simulink model "PMSM_PI_decomposition2018b"  (R2020a)
settings: Solver=ode23tb  StartTime=0.0  StopTime=1  FixedStep=Ts  RelTol=1e-4  EnableMultiTasking=on
InitFcn:
  | Ts = 10e-6;
  | 
  | R = 0.958;
  | Ld = 5.25e-3;
  | Lq = 12e-3;
  | Pn = 4;
  | flux = 0.1827;
undefined symbols (not defined in the file or in its folder): DiscIntNeverNeededParam
libraries: powerlib x4, simulink x1
settings Model: Creator=SUN  LastModifiedBy=Lenovo
settings SolverCC: ZeroCrossControl=DisableAll
settings DataIOCC: LimitDataPoints=on  SaveFormat=Array  SignalLoggingSaveFormat=ModelDataLogs  ReturnWorkspaceOutputs=off
settings OptimizationCC: ExpressionDepthLimit=2147483647  InitFltsAndDblsToZero=on  LifeSpan=inf
settings DebuggingCC: UnderspecifiedInitializationDetection=Classic  MergeDetectMultiDrivingBlocksExec=none  SolverPrmCheckMsg=warning  FcnCallInpInsideContextMsg=warning  StateNameClashWarn=warning  SFUnexpectedBacktrackingDiag=warning  SFNoUnconditionalDefaultTransitionDiag=warning  SFExecutionAtInitializationDiag=none  ArithmeticOperatorsInVariantConditions=warning
settings HardwareCC: ProdBitPerPointer=32  ProdBitPerSizeT=32  ProdBitPerPtrDiffT=32  ProdLargestAtomicFloat=None  ProdIntDivRoundTo=Undefined  ProdEndianess=Unspecified  ProdWordSize=32  ProdHWDeviceType=32-bit Generic
settings ModelReferenceCC: PropagateSignalLabelsOutOfModel=off
settings SFSimCC: SimUseLocalCustomCode=off  CustomCodeUndefinedFunction=UseInterfaceOnly
settings RTWCC: RTWUseLocalCustomCode=off
settings CodeAppCC: StateflowObjectComments=on
settings GRTTargetCC: TargetLangStandard=C89/C90 (ANSI)  CombineOutputUpdateFcns=off  GRTInterface=on
settings ConfigComp: CovMetricSettings=dw  CovHtmlReporting=on  CovSaveCumulativeToWorkspaceVar=on  CovSaveSingleToWorkspaceVar=on  CovExternalEMLEnable=off  CovSFcnEnable=off
settings SimscapeCC: SimscapeNormalizeSystem=off

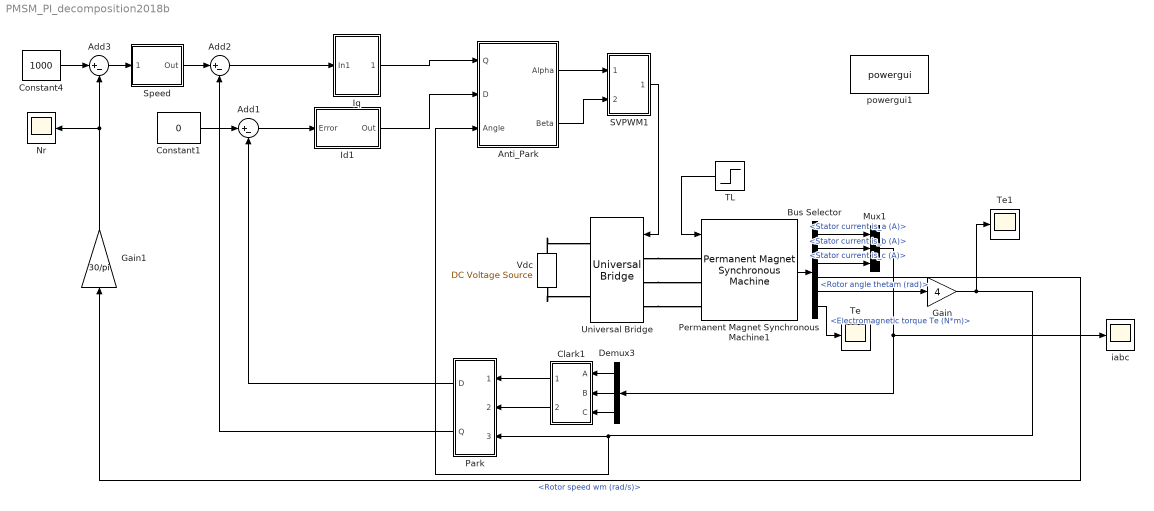
== system PMSM_PI_decomposition2018b ==
  Add1 : Sum  Inputs=|+-
  Add2 : Sum  Inputs=|+-
  Add3 : Sum  Inputs=|+-
  Anti_Park : Subsystem
  Bus Selector : BusSelector  OutputSignals=Stator current is_a (A),Stator current is_b (A),Stator current is_c (A),Rotor speed wm (rad/s),Rotor angle thetam (rad),Electromagnetic torque Te (N*m)
  Clark1 : Subsystem
  Constant1 : Constant  Value=0
  Constant4 : Constant  Value=1000
  Demux3 : Demux  Outputs=3
  Gain : Gain  Gain=4
  Gain1 : Gain  Gain=30/pi
  Id1 : Subsystem  AncestorBlock=|  DialogController=POWERSYS.PowerSysDialog  mask(Discrete PI Controller){Kp=Ld*1100, Ki=R*1100, Par_Limits=[311*0.9*sqrt(1/3) -311*0.9*sqrt(1/3)], Init=0, Ts=Ts}
      | powerlib_extras/Discrete 
      | Control Blocks/Discrete
      | PI Controller
      mask prompts: Kp "Proportional gain (Kp):"; Ki "Integral gain (Ki):"; Par_Limits "Output limits: [ Upper   Lower ]"; Init "Output initial value:"; Ts "Sample time:"
      mask help: This block implements a discrete PI controller.
      mask init:
      | UpperLimit=Par_Limits(1);
      | LowerLimit=Par_Limits(2);
      | power_initmask();
      mask Help: This block is part of a subset of blocks in the Extras library that does not have documentation associated with it, other than the block mask description.
      mask Display: disp('PI');
  "Iq " : Subsystem  mask{Kp=Lq*1100, Ki=R*1100, Init=0, Ts=Ts, max=311*0.9*sqrt(1/3), min=-311*0.9*sqrt(1/3)}
      mask help: This block implement PI Controller
      mask Display: disp('PI')
  Mux1 : Mux  Inputs=3
  Nr : Scope
  Park : Subsystem
  Permanent Magnet Synchronous Machine1 : powerlib/Machines/Permanent Magnet Synchronous Machine  NbPhases=3  FluxDistribution=Sinusoidal  RotorType=Salient-pole  MechanicalLoad=Torque Tm  PresetModel=No  ShowDetailedParameters=on  MeasurementBus=off  Resistance=0.958  Inductance=8.5e-3  dqInductances=[5.25e-3,12e-3]  La=0.000835  MachineConstant=Flux linkage established by magnets (V.s)  Flux=0.1827  VoltageCst=132.5525  TorqueCst=1.0962  Flat=120  Mechanical=[0.003 0.008 4]  PolePairs=3  InitialConditions=[0,0, 0,0]  InitialConditions5ph=[0 0 0 0 0 0]  RefAngle=Aligned with phase A axis (original Park)  IterativeDiscreteModel=Trapezoidal non iterative  TsBlock=-1  TsPowergui=0
  SVPWM1 : Subsystem
  Speed : Subsystem  AncestorBlock=|  DialogController=POWERSYS.PowerSysDialog  mask(Discrete PI Controller){Kpw=0.14, Kiw=0.14*50, Ba=0.013, Par_Limits=[30 -30], Init=0, Ts=Ts}
      | powerlib_extras/Discrete 
      | Control Blocks/Discrete
      | PI Controller
      mask prompts: Kpw "Proportional gain (Kp):"; Kiw "Integral gain (Ki):"; Ba "feedback gain (Ba)"; Par_Limits "Output limits: [ Upper   Lower ]"; Init "Output initial value:"; Ts "Sample time:"
      mask help: This block implements a discrete PI controller.
      mask init:
      | UpperLimit=Par_Limits(1);
      | LowerLimit=Par_Limits(2);
      | power_initmask();
      mask Help: This block is part of a subset of blocks in the Extras library that does not have documentation associated with it, other than the block mask description.
      mask Display: disp('PI');
  TL : Step  Time=0.2  After=10  SampleTime=0
  Te : Scope
  Te1 : Scope
  Universal Bridge : powerlib/Power Electronics/Universal Bridge  Arms=3  SnubberResistance=1e5  SnubberCapacitance=inf  Device=IGBT / Diodes  Ron=1e-3  Lon=0  ForwardVoltages="[  0  0  ]"  ForwardVoltage=0  GTOparameters=[ 10e-6 , 20e-6 ]  IGBTparameters=[ 1e-6 , 2e-6 ]  Measurements=None  Measurements_2=None  converterType=Rectifier
  Vdc : powerlib/Electrical Sources/DC Voltage Source  Amplitude=311  Measurements=None
  iabc : Scope
  powergui1 : powerlib/powergui  Priority=1  SimulationMode=Continuous  SampleTime=50e-6  frequency=60  Iterations=50  frequencyindice=0  Pbase=100e6  ErrMax=1e-4  UnitsV=kV  UnitsW=MW  buscounter=0  FunctionMessages=off  echomessages=off  EnableUseOfTLC=off  CurrentSourceSwitches=off  DisableSnubberDevices=off  DisableRonSwitches=off  DisableVfSwitches=off  DisplayEquations=off  AutomaticDiscreteSolvers=off  SolverType=Tustin/Backward Euler (TBE)  Interpol=off  ExternalGateDelay=off  methode=off  Ts=100  x0status=blocks  SPID=on  SwTol=0  HookPort=off  NonlinearTolerance=1e-4  nMaxIteration=100  ContinueOnMaxIteration=off  RestoreLinks=warning  ResistiveCurrentMeasurement=off  Frange=[0:2:500]  Ylog=off  Xlog=on  ShowGrid=off  save=off  variable=ZData  structure=0  ZoomFFT=off  StartTime=0.0  cycles=1  DisplayStyle=1  fundamental=60  FreqAxis=off  MaxFrequency=1000  frequencyindicesteady=1  RmsSteady=1  display=off
  wires:
  TL/1 -> Permanent Magnet Synchronous Machine1/1
  Add3/1 -> Speed/1(Error)
  Constant4/1 -> Add3/1
  Constant1/1 -> Add1/1
  Add1/1 -> Id1/1(Error)
  Gain1/1 -> Add3/2, Nr/1
  Id1/1(Out) -> Anti_Park/2(D)
  Speed/1(Out) -> Add2/1
  Add2/1 -> "Iq "/1(In1)
  "Iq "/1(Out1) -> Anti_Park/1(Q)
  Gain/1 -> Te1/1, Park/3(Angle), Anti_Park/3(Angle)
  SVPWM1/1(pulse1) -> Universal Bridge/1
  Anti_Park/1(Alpha) -> SVPWM1/1(Ualpha)
  Demux3/1 -> Clark1/1(A)
  Park/1(D) -> Add1/2
  Park/2(Q) -> Add2/2
  Anti_Park/2(Beta) -> SVPWM1/2(Ubeta)
  Demux3/2 -> Clark1/2(B)
  Demux3/3 -> Clark1/3(C)
  Clark1/1(Alpha) -> Park/1(Alpha)
  Clark1/2(Beta) -> Park/2(Beta)
  Bus Selector/3 -> Mux1/3  "<Stator current is_c (A)>"
  Bus Selector/2 -> Mux1/2  "<Stator current is_b (A)>"
  Bus Selector/1 -> Mux1/1  "<Stator current is_a (A)>"
  Mux1/1 -> iabc/1, Demux3/1
  Permanent Magnet Synchronous Machine1/1 -> Bus Selector/1
  Bus Selector/5 -> Gain/1  "<Rotor angle thetam (rad)>"
  Bus Selector/4 -> Gain1/1  "<Rotor speed wm (rad/s)>"
  Bus Selector/6 -> Te/1  "<Electromagnetic torque Te (N*m)>"
  connections:
  Universal Bridge/LConn1 -- Permanent Magnet Synchronous Machine1/LConn1
  Universal Bridge/LConn2 -- Permanent Magnet Synchronous Machine1/LConn2
  Universal Bridge/LConn3 -- Permanent Magnet Synchronous Machine1/LConn3
  Vdc/RConn1 -- Universal Bridge/RConn1
  Vdc/LConn1 -- Universal Bridge/RConn2

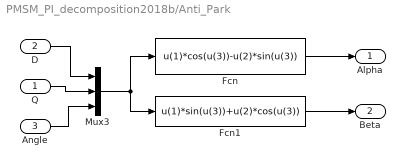
== system PMSM_PI_decomposition2018b/Anti_Park ==
  Q : Inport
  D : Inport  Port=2
  Angle : Inport  Port=3
  Fcn : Fcn  Expr=u(1)*cos(u(3))-u(2)*sin(u(3))
  Fcn1 : Fcn  Expr=u(1)*sin(u(3))+u(2)*cos(u(3))
  Mux3 : Mux  Inputs=3
  Alpha : Outport  VectorParamsAs1DForOutWhenUnconnected=off
  Beta : Outport  Port=2  VectorParamsAs1DForOutWhenUnconnected=off
  wires:
  Angle/1 -> Mux3/3
  Fcn1/1 -> Beta/1
  Mux3/1 -> Fcn1/1, Fcn/1
  Fcn/1 -> Alpha/1
  D/1 -> Mux3/1
  Q/1 -> Mux3/2

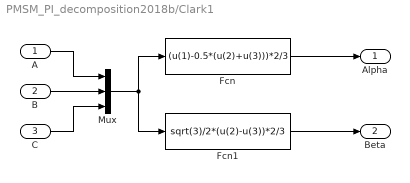
== system PMSM_PI_decomposition2018b/Clark1 ==
  A : Inport
  B : Inport  Port=2
  C : Inport  Port=3
  Fcn : Fcn  Expr=(u(1)-0.5*(u(2)+u(3)))*2/3
  Fcn1 : Fcn  Expr=sqrt(3)/2*(u(2)-u(3))*2/3
  Mux : Mux  Inputs=3
  Alpha : Outport  VectorParamsAs1DForOutWhenUnconnected=off
  Beta : Outport  Port=2  VectorParamsAs1DForOutWhenUnconnected=off
  wires:
  B/1 -> Mux/2
  Mux/1 -> Fcn1/1, Fcn/1
  Fcn1/1 -> Beta/1
  Fcn/1 -> Alpha/1
  C/1 -> Mux/3
  A/1 -> Mux/1

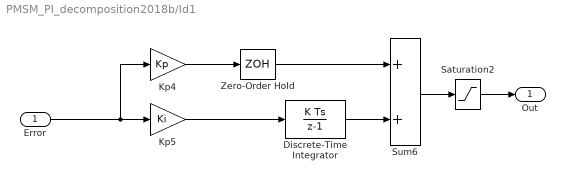
== system PMSM_PI_decomposition2018b/Id1 ==
  Error : Inport  SampleTime=Ts
  Discrete-Time Integrator : DiscreteIntegrator  InitialCondition=Init  SampleTime=Ts  LimitOutput=on  UpperSaturationLimit=UpperLimit  LowerSaturationLimit=LowerLimit  ICPrevOutput=DiscIntNeverNeededParam  ICPrevScaledInput=DiscIntNeverNeededParam
  Kp4 : Gain  Gain=Kp  SaturateOnIntegerOverflow=on  SampleTime=Ts  OutDataTypeStr=Inherit: Same as input  ParamDataTypeStr=Inherit: Same as input
  Kp5 : Gain  Gain=Ki  SaturateOnIntegerOverflow=on  SampleTime=Ts  OutDataTypeStr=Inherit: Same as input  ParamDataTypeStr=Inherit: Same as input
  Saturation2 : Saturate  UpperLimit=UpperLimit  LowerLimit=LowerLimit  SampleTime=Ts
  Sum6 : Sum  InputSameDT=on  SaturateOnIntegerOverflow=on  SampleTime=Ts  OutDataTypeStr=Inherit: Same as first input
  Zero-Order Hold : ZeroOrderHold  SampleTime=Ts
  Out : Outport  SampleTime=Ts  InitialOutput=0  VectorParamsAs1DForOutWhenUnconnected=off
  wires:
  Zero-Order Hold/1 -> Sum6/1
  Saturation2/1 -> Out/1
  Discrete-Time Integrator/1 -> Sum6/2
  Kp4/1 -> Zero-Order Hold/1
  Kp5/1 -> Discrete-Time Integrator/1
  Sum6/1 -> Saturation2/1
  Error/1 -> Kp5/1, Kp4/1

== system PMSM_PI_decomposition2018b/Iq  ==
  In1 : Inport
  Add : Sum
  Discrete-Time Integrator : DiscreteIntegrator  InitialCondition=Init  SampleTime=Ts  LimitOutput=on  UpperSaturationLimit=max  LowerSaturationLimit=min  ICPrevOutput=DiscIntNeverNeededParam  ICPrevScaledInput=DiscIntNeverNeededParam
  Gain : Gain  Gain=Kp
  Gain3 : Gain  Gain=Ki
  Saturation : Saturate  UpperLimit=max  LowerLimit=min
  Zero-Order Hold : ZeroOrderHold  SampleTime=Ts
  Out1 : Outport  VectorParamsAs1DForOutWhenUnconnected=off
  wires:
  Saturation/1 -> Out1/1
  In1/1 -> Gain/1, Gain3/1
  Zero-Order Hold/1 -> Add/1
  Gain/1 -> Zero-Order Hold/1
  Add/1 -> Saturation/1
  Discrete-Time Integrator/1 -> Add/2
  Gain3/1 -> Discrete-Time Integrator/1

== system PMSM_PI_decomposition2018b/Park ==
  Alpha : Inport
  Beta : Inport  Port=2
  Angle : Inport  Port=3
  Fcn : Fcn  Expr=u(1)*cos(u(3))+u(2)*sin(u(3))
  Fcn1 : Fcn  Expr=u(2)*cos(u(3))-u(1)*sin(u(3))
  Mux2 : Mux  Inputs=3
  D : Outport  VectorParamsAs1DForOutWhenUnconnected=off
  Q : Outport  Port=2  VectorParamsAs1DForOutWhenUnconnected=off
  wires:
  Beta/1 -> Mux2/2
  Mux2/1 -> Fcn1/1, Fcn/1
  Angle/1 -> Mux2/3
  Alpha/1 -> Mux2/1
  Fcn1/1 -> Q/1
  Fcn/1 -> D/1

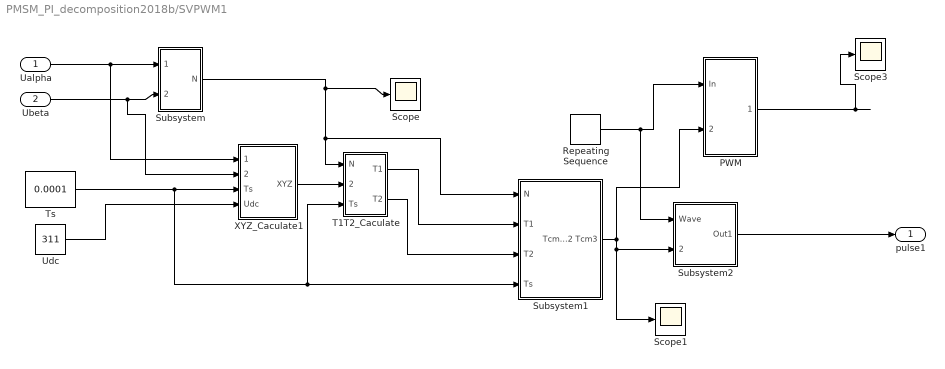
== system PMSM_PI_decomposition2018b/SVPWM1 ==
  Ualpha : Inport
  Ubeta : Inport  Port=2
  PWM : Subsystem
  Repeating Sequence : simulink/Sources/Repeating Sequence  rep_seq_t=[0 0.00005 0.0001]  rep_seq_y=[0 0.00005 0]
  Scope : Scope
  Scope1 : Scope
  Scope3 : Scope
  Subsystem : Subsystem
  Subsystem1 : Subsystem
  Subsystem2 : Subsystem
  T1T2_Caculate : Subsystem
  Ts : Constant  Value=0.0001
  Udc : Constant  Value=311
  XYZ_Caculate1 : Subsystem
  pulse1 : Outport  VectorParamsAs1DForOutWhenUnconnected=off
  wires:
  T1T2_Caculate/1(T1) -> Subsystem1/2(T1)
  Ts/1 -> XYZ_Caculate1/3(Ts), T1T2_Caculate/3(Ts), Subsystem1/4(Ts)
  Udc/1 -> XYZ_Caculate1/4(Udc)
  Subsystem/1(N) -> Scope/1, T1T2_Caculate/1(N), Subsystem1/1(N)
  T1T2_Caculate/2(T2) -> Subsystem1/3(T2)
  XYZ_Caculate1/1("XYZ ") -> T1T2_Caculate/2(XYZ)
  Ualpha/1 -> XYZ_Caculate1/1(Ualpha), Subsystem/1(Ualpha)
  Ubeta/1 -> XYZ_Caculate1/2(Ubeta), Subsystem/2(Ubeta)
  Subsystem1/1(Tcm1 Tcm2 Tcm3) -> Scope1/1, Subsystem2/2(Tcm123), PWM/2(Tcm123)
  Repeating Sequence/1 -> Subsystem2/1(Wave), PWM/1(In)
  PWM/1(PWM) -> Scope3/1
  Subsystem2/1(Out1) -> pulse1/1

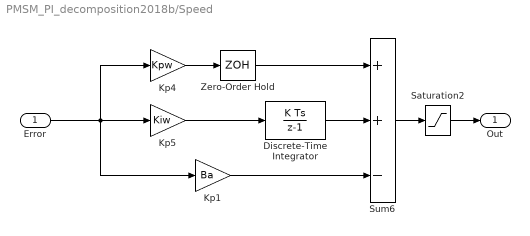
== system PMSM_PI_decomposition2018b/Speed ==
  Error : Inport  SampleTime=Ts
  Discrete-Time Integrator : DiscreteIntegrator  InitialCondition=Init  SampleTime=Ts  LimitOutput=on  UpperSaturationLimit=UpperLimit  LowerSaturationLimit=LowerLimit  ICPrevOutput=DiscIntNeverNeededParam  ICPrevScaledInput=DiscIntNeverNeededParam
  Kp1 : Gain  Gain=Ba  SaturateOnIntegerOverflow=on  SampleTime=Ts  OutDataTypeStr=Inherit: Same as input  ParamDataTypeStr=Inherit: Same as input
  Kp4 : Gain  Gain=Kpw  SaturateOnIntegerOverflow=on  SampleTime=Ts  OutDataTypeStr=Inherit: Same as input  ParamDataTypeStr=Inherit: Same as input
  Kp5 : Gain  Gain=Kiw  SaturateOnIntegerOverflow=on  SampleTime=Ts  OutDataTypeStr=Inherit: Same as input  ParamDataTypeStr=Inherit: Same as input
  Saturation2 : Saturate  UpperLimit=UpperLimit  LowerLimit=LowerLimit  SampleTime=Ts
  Sum6 : Sum  Inputs=++-  InputSameDT=on  SaturateOnIntegerOverflow=on  SampleTime=Ts  OutDataTypeStr=Inherit: Same as first input
  Zero-Order Hold : ZeroOrderHold  SampleTime=Ts
  Out : Outport  SampleTime=Ts  InitialOutput=0  VectorParamsAs1DForOutWhenUnconnected=off
  wires:
  Error/1 -> Kp1/1, Kp5/1, Kp4/1
  Zero-Order Hold/1 -> Sum6/1
  Saturation2/1 -> Out/1
  Discrete-Time Integrator/1 -> Sum6/2
  Kp4/1 -> Zero-Order Hold/1
  Kp5/1 -> Discrete-Time Integrator/1
  Sum6/1 -> Saturation2/1
  Kp1/1 -> Sum6/3

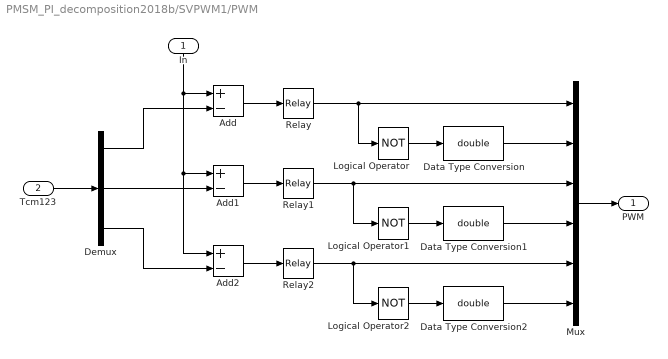
== system PMSM_PI_decomposition2018b/SVPWM1/PWM ==
  In : Inport
  Tcm123 : Inport  Port=2
  Add : Sum  Inputs=+-
  Add1 : Sum  Inputs=+-
  Add2 : Sum  Inputs=+-
  Data Type Conversion : DataTypeConversion  OutDataTypeStr=double
  Data Type Conversion1 : DataTypeConversion  OutDataTypeStr=double
  Data Type Conversion2 : DataTypeConversion  OutDataTypeStr=double
  Demux : Demux  Outputs=3
  Logical Operator : Logic  Operator=NOT  AllPortsSameDT=off  OutDataTypeStr=boolean
  Logical Operator1 : Logic  Operator=NOT  AllPortsSameDT=off  OutDataTypeStr=boolean
  Logical Operator2 : Logic  Operator=NOT  AllPortsSameDT=off  OutDataTypeStr=boolean
  Mux : Mux  Inputs=6
  Relay : Relay  OffSwitchValue=-eps
  Relay1 : Relay  OffSwitchValue=-eps
  Relay2 : Relay  OffSwitchValue=-eps
  PWM : Outport  VectorParamsAs1DForOutWhenUnconnected=off
  wires:
  Demux/3 -> Add2/2
  Demux/2 -> Add1/2
  Demux/1 -> Add/2
  Relay2/1 -> Mux/5, Logical Operator2/1
  Relay1/1 -> Mux/3, Logical Operator1/1
  Relay/1 -> Logical Operator/1, Mux/1
  Mux/1 -> PWM/1
  Data Type Conversion/1 -> Mux/2
  Data Type Conversion1/1 -> Mux/4
  Data Type Conversion2/1 -> Mux/6
  Logical Operator2/1 -> Data Type Conversion2/1
  Logical Operator1/1 -> Data Type Conversion1/1
  Logical Operator/1 -> Data Type Conversion/1
  Add1/1 -> Relay1/1
  Add2/1 -> Relay2/1
  Add/1 -> Relay/1
  In/1 -> Add/1, Add2/1, Add1/1
  Tcm123/1 -> Demux/1

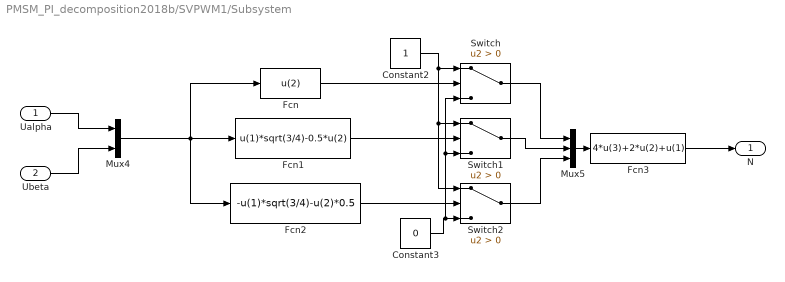
== system PMSM_PI_decomposition2018b/SVPWM1/Subsystem ==
  Ualpha : Inport
  Ubeta : Inport  Port=2
  Constant2 : Constant
  Constant3 : Constant  Value=0
  Fcn : Fcn  Expr=u(2)
  Fcn1 : Fcn  Expr=u(1)*sqrt(3/4)-0.5*u(2)
  Fcn2 : Fcn  Expr=-u(1)*sqrt(3/4)-u(2)*0.5
  Fcn3 : Fcn  Expr=4*u(3)+2*u(2)+u(1)
  Mux4 : Mux  Inputs=2
  Mux5 : Mux  Inputs=3
  Switch : Switch  Criteria=u2 > Threshold
  Switch1 : Switch  Criteria=u2 > Threshold
  Switch2 : Switch  Criteria=u2 > Threshold
  N : Outport  VectorParamsAs1DForOutWhenUnconnected=off
  wires:
  Switch/1 -> Mux5/1
  Ualpha/1 -> Mux4/1
  Constant2/1 -> Switch2/1, Switch1/1, Switch/1
  Mux4/1 -> Fcn/1, Fcn2/1, Fcn1/1
  Fcn2/1 -> Switch2/2
  Ubeta/1 -> Mux4/2
  Fcn3/1 -> N/1
  Constant3/1 -> Switch/3, Switch1/3, Switch2/3
  Fcn/1 -> Switch/2
  Switch2/1 -> Mux5/3
  Fcn1/1 -> Switch1/2
  Switch1/1 -> Mux5/2
  Mux5/1 -> Fcn3/1

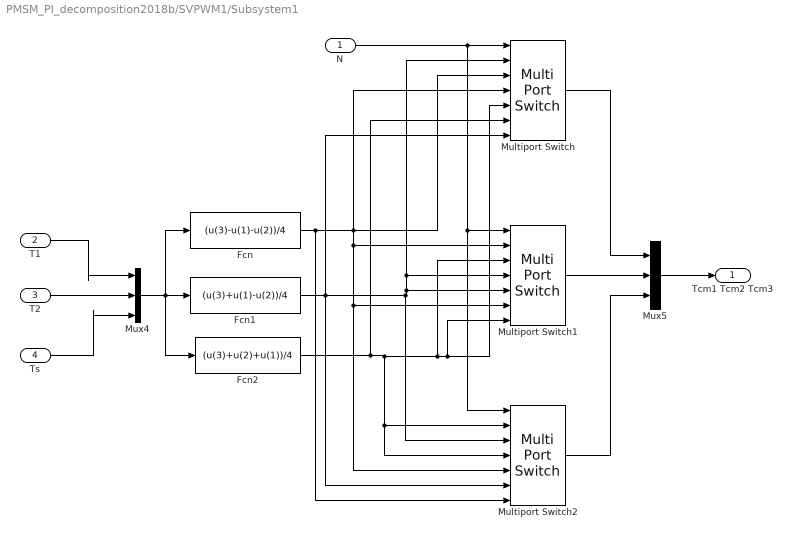
== system PMSM_PI_decomposition2018b/SVPWM1/Subsystem1 ==
  N : Inport
  T1 : Inport  Port=2
  T2 : Inport  Port=3
  Ts : Inport  Port=4
  Fcn : Fcn  Expr=(u(3)-u(1)-u(2))/4
  Fcn1 : Fcn  Expr=(u(3)+u(1)-u(2))/4
  Fcn2 : Fcn  Expr=(u(3)+u(2)+u(1))/4
  Multiport Switch : MultiPortSwitch  Inputs=6
  Multiport Switch1 : MultiPortSwitch  Inputs=6
  Multiport Switch2 : MultiPortSwitch  Inputs=6
  Mux4 : Mux  Inputs=3
  Mux5 : Mux  Inputs=3
  Tcm1 Tcm2 Tcm3 : Outport  VectorParamsAs1DForOutWhenUnconnected=off
  wires:
  T2/1 -> Mux4/2
  N/1 -> Multiport Switch2/1, Multiport Switch1/1, Multiport Switch/1
  Mux5/1 -> Tcm1 Tcm2 Tcm3/1
  T1/1 -> Mux4/1
  Fcn1/1 -> Multiport Switch/7, Multiport Switch2/6, Multiport Switch2/3, Multiport Switch1/5, Multiport Switch1/4, Multiport Switch/2
  Mux4/1 -> Fcn2/1, Fcn1/1, Fcn/1
  Multiport Switch2/1 -> Mux5/3
  Fcn/1 -> Multiport Switch2/7, Multiport Switch1/6, Multiport Switch2/5, Multiport Switch1/2, Multiport Switch/3, Multiport Switch/4
  Multiport Switch1/1 -> Mux5/2
  Fcn2/1 -> Multiport Switch/6, Multiport Switch1/7, Multiport Switch/5, Multiport Switch1/3, Multiport Switch2/4, Multiport Switch2/2
  Ts/1 -> Mux4/3
  Multiport Switch/1 -> Mux5/1

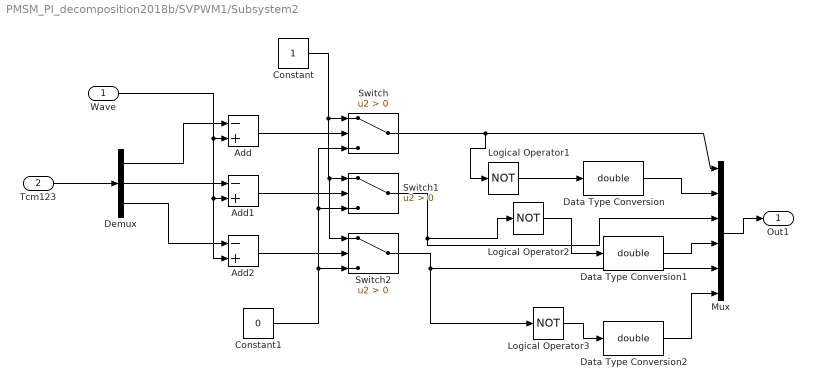
== system PMSM_PI_decomposition2018b/SVPWM1/Subsystem2 ==
  Wave : Inport
  Tcm123 : Inport  Port=2
  Add : Sum  Inputs=-+
  Add1 : Sum  Inputs=-+
  Add2 : Sum  Inputs=-+
  Constant : Constant
  Constant1 : Constant  Value=0
  Data Type Conversion : DataTypeConversion  OutDataTypeStr=double
  Data Type Conversion1 : DataTypeConversion  OutDataTypeStr=double
  Data Type Conversion2 : DataTypeConversion  OutDataTypeStr=double
  Demux : Demux  Outputs=3
  Logical Operator1 : Logic  Operator=NOT  AllPortsSameDT=off  OutDataTypeStr=boolean
  Logical Operator2 : Logic  Operator=NOT  AllPortsSameDT=off  OutDataTypeStr=boolean
  Logical Operator3 : Logic  Operator=NOT  AllPortsSameDT=off  OutDataTypeStr=boolean
  Mux : Mux  Inputs=6
  Switch : Switch  Criteria=u2 > Threshold
  Switch1 : Switch  Criteria=u2 > Threshold
  Switch2 : Switch  Criteria=u2 > Threshold
  Out1 : Outport  VectorParamsAs1DForOutWhenUnconnected=off
  wires:
  Add2/1 -> Switch2/2
  Add1/1 -> Switch1/2
  Constant/1 -> Switch2/1, Switch1/1, Switch/1
  Switch/1 -> Logical Operator1/1, Mux/1
  Wave/1 -> Add2/2, Add1/2, Add/2
  Demux/3 -> Add2/1
  Constant1/1 -> Switch2/3, Switch1/3, Switch/3
  Add/1 -> Switch/2
  Switch1/1 -> Mux/3, Logical Operator2/1
  Switch2/1 -> Mux/5, Logical Operator3/1
  Demux/1 -> Add/1
  Tcm123/1 -> Demux/1
  Demux/2 -> Add1/1
  Mux/1 -> Out1/1
  Logical Operator1/1 -> Data Type Conversion/1
  Data Type Conversion/1 -> Mux/2
  Data Type Conversion1/1 -> Mux/4
  Logical Operator2/1 -> Data Type Conversion1/1
  Data Type Conversion2/1 -> Mux/6
  Logical Operator3/1 -> Data Type Conversion2/1

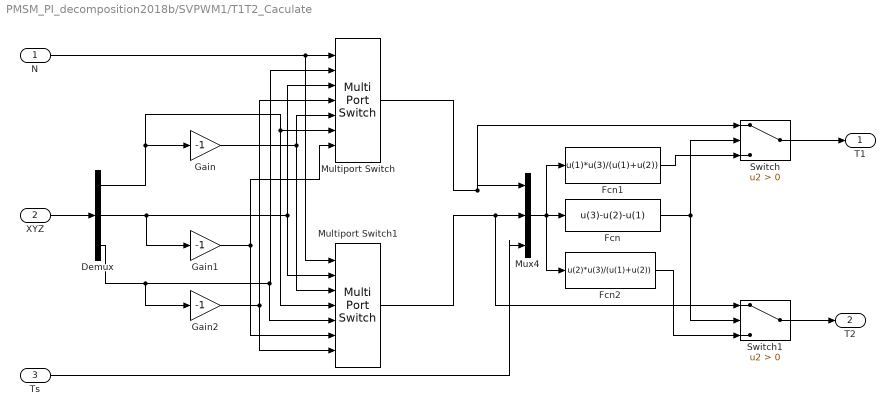
== system PMSM_PI_decomposition2018b/SVPWM1/T1T2_Caculate ==
  N : Inport
  XYZ : Inport  Port=2
  Ts : Inport  Port=3
  Demux : Demux  Outputs=3
  Fcn : Fcn  Expr=u(3)-u(2)-u(1)
  Fcn1 : Fcn  Expr=u(1)*u(3)/(u(1)+u(2))
  Fcn2 : Fcn  Expr=u(2)*u(3)/(u(1)+u(2))
  Gain : Gain  Gain=-1
  Gain1 : Gain  Gain=-1
  Gain2 : Gain  Gain=-1
  Multiport Switch : MultiPortSwitch  Inputs=6
  Multiport Switch1 : MultiPortSwitch  Inputs=6
  Mux4 : Mux  Inputs=3
  Switch : Switch  Criteria=u2 > Threshold
  Switch1 : Switch  Criteria=u2 > Threshold
  T1 : Outport  VectorParamsAs1DForOutWhenUnconnected=off
  T2 : Outport  Port=2  VectorParamsAs1DForOutWhenUnconnected=off
  wires:
  Gain1/1 -> Multiport Switch/7, Multiport Switch1/6
  Fcn2/1 -> Switch1/3
  Demux/2 -> Gain1/1, Multiport Switch/3, Multiport Switch1/2
  Demux/3 -> Multiport Switch1/5, Multiport Switch/2, Gain2/1
  N/1 -> Multiport Switch1/1, Multiport Switch/1
  Demux/1 -> Gain/1, Multiport Switch/6, Multiport Switch1/4
  Mux4/1 -> Fcn2/1, Fcn1/1, Fcn/1
  XYZ/1 -> Demux/1
  Gain/1 -> Multiport Switch1/3, Multiport Switch/5
  Fcn/1 -> Switch1/2, Switch/2
  Multiport Switch1/1 -> Switch1/1, Mux4/2
  Fcn1/1 -> Switch/3
  Multiport Switch/1 -> Switch/1, Mux4/1
  Gain2/1 -> Multiport Switch1/7, Multiport Switch/4
  Switch1/1 -> T2/1
  Ts/1 -> Mux4/3
  Switch/1 -> T1/1

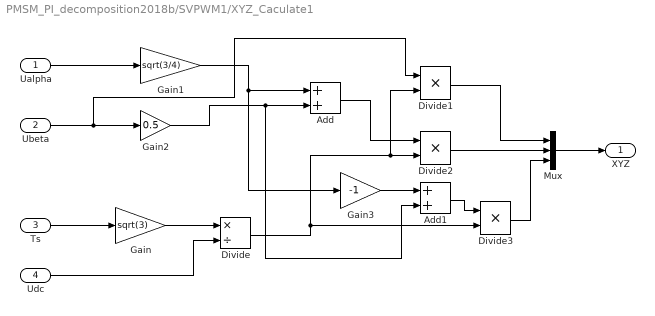
== system PMSM_PI_decomposition2018b/SVPWM1/XYZ_Caculate1 ==
  Ualpha : Inport
  Ubeta : Inport  Port=2
  Ts : Inport  Port=3
  Udc : Inport  Port=4
  Add : Sum
  Add1 : Sum
  Divide : Product  Inputs=*/
  Divide1 : Product  Inputs=**
  Divide2 : Product  Inputs=**
  Divide3 : Product  Inputs=**
  Gain : Gain  Gain=sqrt(3)
  Gain1 : Gain  Gain=sqrt(3/4)
  Gain2 : Gain  Gain=0.5
  Gain3 : Gain  Gain=-1
  Mux : Mux  Inputs=3
  "XYZ " : Outport  VectorParamsAs1DForOutWhenUnconnected=off
  wires:
  Mux/1 -> "XYZ "/1
  Divide2/1 -> Mux/2
  Divide1/1 -> Mux/1
  Gain/1 -> Divide/1
  Udc/1 -> Divide/2
  Ualpha/1 -> Gain1/1
  Add/1 -> Divide2/1
  Divide/1 -> Divide3/2, Divide2/2, Divide1/2
  Gain3/1 -> Add1/1
  Ubeta/1 -> Divide1/1, Gain2/1
  Gain1/1 -> Add/1, Gain3/1
  Gain2/1 -> Add/2, Add1/2
  Ts/1 -> Gain/1
  Add1/1 -> Divide3/1
  Divide3/1 -> Mux/3
